simulink model "contador"  (R2013a)
settings: Solver=ode4  StartTime=0.0  StopTime=1000  FixedStep=0.05  RelTol=1e-3
libraries: instrumentlib x1
settings Model: Creator=Administrator  LastModifiedBy=Administrator

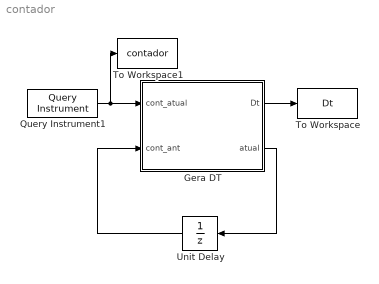
== system contador ==
  Gera DT : MATLAB Function  TreatAsAtomicUnit=on
  Query Instrument1 : instrumentlib/Query Instrument  sampleTime=.05  isWorkspaceObject=off  timeout=5  inputBufferSize=200  protocol=Serial  serialPort=COM3  baudRate=115200  gpibVendor=Advantech  boardIndex=0  primaryAddress=1  secondaryAddress=0  visaVendor=Agilent  visaSerialPort=0  chassisIndex=0  logicalAddress=0  tcpRemoteHost='127.0.0.1'  tcpRemotePort=4500  udpRemoteHost='127.0.0.1'  udpRemotePort=9090  visaTCPBoardIndex=0  visaTCPRemoteHost='127.0.0.1'  usbBoardIndex=0  usbManufID=0  usbModelCode=0  usbSerialNumber=0  initAction=None  initCommand='DATA:SOURCE CH1'  initFunction=get  queryCommand='%'  responseFormat=ASCII  asciiFormatting='%d'  precision=16-bit integer  byteOrder=Little endian  valuesToRead=18  removeBytes=on  afterOutputAction=Repeat query for new data  enableFrames=on  frameSize=1
  To Workspace : ToWorkspace  VariableName=Dt  SampleTime=-1
  To Workspace1 : ToWorkspace  VariableName=contador  SampleTime=-1
  Unit Delay : UnitDelay  InitialCondition=44444  SampleTime=0.05
  wires:
  Query Instrument1/1 -> To Workspace1/1, Gera DT/1(cont_atual)
  Unit Delay/1 -> Gera DT/2(cont_ant)
  Gera DT/2(atual) -> Unit Delay/1
  Gera DT/1(Dt) -> To Workspace/1

== matlab function contador/Gera DT ==
  data: cont_atual input; Dt output; cont_ant input; atual output
function [Dt, atual]  = gera_dt(cont_atual, cont_ant)
%#codegen

if (cont_ant > 44443)
    Dt = 0;
    atual = cont_atual;
else
    if (cont_atual<=cont_ant)
        Dt = (10000-cont_ant) + cont_atual;
        Dt = Dt * 0.0001;
        atual = cont_atual;
    else
        Dt = cont_atual - cont_ant;
        Dt = Dt * 0.0001;
        atual = cont_atual;
    end
end
